simulink model "torque_model_validation_2"  (R2023b)
settings: Solver=VariableStepAuto  StartTime=0.0  StopTime=20  RelTol=1e-3  EnableMultiTasking=on
settings Model: SimulationMode=external  ExtModeTrigDuration=10  Creator=kiraa  LastModifiedBy=kiraa
settings OptimizationCC: EnhancedBackFolding=on  PassReuseOutputArgsThreshold=0  MaxStackSize=64  OptimizeBlockOrder=speed  DifferentSizesBufferReuse=on  OptimizationCustomize=off
settings DebuggingCC: ParameterTunabilityLossMsg=error
settings HardwareCC: ProdBitPerPointer=32  ProdBitPerSizeT=32  ProdBitPerPtrDiffT=32  ProdLargestAtomicInteger=Long  ProdLargestAtomicFloat=Double  ProdWordSize=32  ProdLongLongMode=on  ProdHWDeviceType=ARM Compatible->ARM Cortex
settings SFSimCC: MATLABDynamicMemAlloc=off
settings RTWCC: Toolchain=GNU Tools for ARM Embedded Processors
settings CodeAppCC: ForceParamTrailComments=on  OperatorAnnotations=on
settings GRTTargetCC: TargetLangStandard=C89/C90 (ANSI)

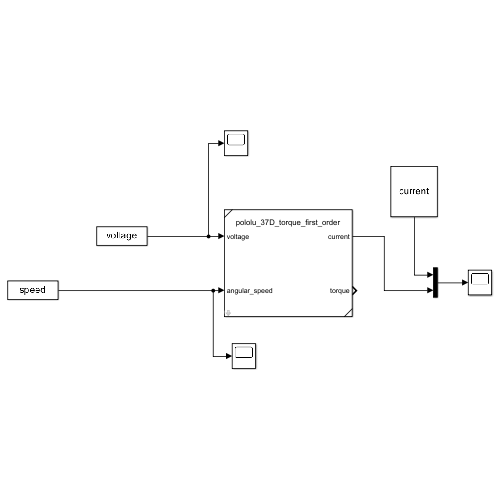
[thumbnail: Simulink's stored preview of the top-level diagram]
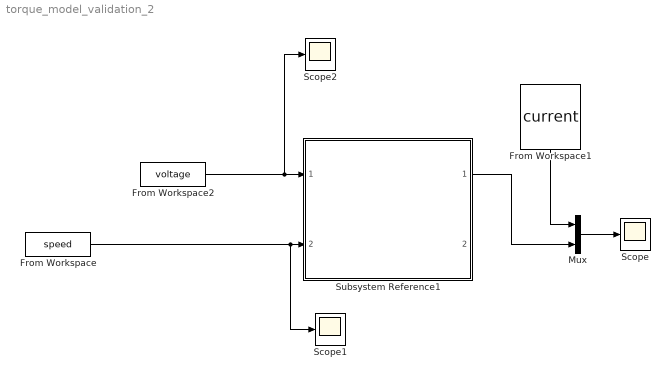
== system torque_model_validation_2 ==
  From Workspace : FromWorkspace  VariableName=speed
  From Workspace1 : FromWorkspace  VariableName=current
  From Workspace2 : FromWorkspace  VariableName=voltage
  Mux : Mux  Inputs=2
  Scope : Scope
  Scope1 : Scope
  Scope2 : Scope
  Subsystem Reference1 : Subsystem  ReferencedSubsystem=pololu_37D_torque_first_order  L=2.3e-3  R=3.4  K=1.335
  wires:
  From Workspace1/1 -> Mux/1
  From Workspace2/1 -> Scope2/1, Subsystem Reference1/1
  Subsystem Reference1/1 -> Mux/2
  Mux/1 -> Scope/1
  From Workspace/1 -> Scope1/1, Subsystem Reference1/2
